simulink model "sim_first_order"  (R2019b)
settings: Solver=VariableStepAuto  StartTime=0.0  StopTime=10.0  RelTol=1e-3
values from neighbouring files (symbols this model uses):
  alpha1 = 0.1853    [single_pool.m]
  tau1 = 0.5    [single_pool.m]
settings Model: Creator=bas  LastModifiedBy=bas
settings DataIOCC: ReturnWorkspaceOutputs=off

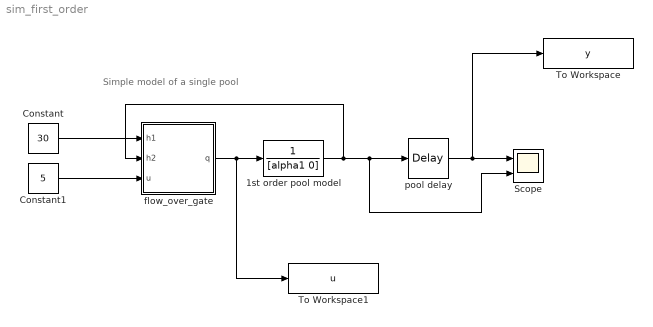
== system sim_first_order ==
  note: Simple model of a single pool
  1st order pool model : TransferFcn  Denominator=[alpha1 0]
  Constant : Constant  Value=30
  Constant1 : Constant  Value=5
  Scope : Scope  NumInputPorts=2
  To Workspace : ToWorkspace  VariableName=y  SaveFormat=Timeseries  SampleTime=-1
  To Workspace1 : ToWorkspace  VariableName=u  SaveFormat=Timeseries  SampleTime=-1
  flow_over_gate : MATLAB Function  TreatAsAtomicUnit=on
  pool delay : TransportDelay  DelayTime=tau1
  wires:
  1st order pool model/1 -> flow_over_gate/2(h2), Scope/2, pool delay/1
  pool delay/1 -> To Workspace/1, Scope/1
  Constant/1 -> flow_over_gate/1(h1)
  Constant1/1 -> flow_over_gate/3(u)
  flow_over_gate/1(q) -> To Workspace1/1, 1st order pool model/1

== matlab function sim_first_order/flow_over_gate ==
  data: h1 input; h2 input; u input; q output
function q = fcn(h1, h2, u)
    % u     : servo 0-255 (step)
    % h1    : height before gate (cm)
    % h2    : height after gate (cm)
    
    % TODO: use real values
     
    %MAX_OPENING = 17; % (cm)
    
    %gate_opening = u/255 * MAX_OPENING;
    
    % need to assume h1 > h2
    if h2 > h1
        q = 0;
    else
        q = 0.05 * u * sqrt(h1-h2);
    end
